simulink model "IntecoPhysicalOriginal"  (R2020b)
settings: Solver=ode5  StartTime=0.0  StopTime=9999  FixedStep=0.01  RelTol=1e-3  AbsTol=1e-6
libraries: simulink x2
settings Model: SimulationMode=external  ExtModeTrigDuration=12000  ExtModeTrigLevel=0.400000  Creator=jims  LastModifiedBy=Mark
settings SolverCC: AutoScaleAbsTol=off
settings DataIOCC: ExternalInput=[]  InitialState=[]  MaxDataPoints=5000  SaveFormat=Array  SignalLoggingSaveFormat=ModelDataLogs  SaveOutput=off  SaveTime=off  ReturnWorkspaceOutputs=off  SignalLoggingName=sigsOut
settings OptimizationCC: BooleanDataType=off  ExpressionDepthLimit=2147483647  InitFltsAndDblsToZero=on
settings DebuggingCC: SaveWithParameterizedLinksMsg=none  UnderspecifiedInitializationDetection=Classic  MergeDetectMultiDrivingBlocksExec=none  SignalResolutionControl=TryResolveAllWithWarning  MultiTaskDSMMsg=warning  MultiTaskCondExecSysMsg=none  IntegerOverflowMsg=none  FcnCallInpInsideContextMsg=warning  StateNameClashWarn=warning  SFUnexpectedBacktrackingDiag=warning  SFNoUnconditionalDefaultTransitionDiag=warning  SFExecutionAtInitializationDiag=none  IntegerSaturationMsg=none  ArithmeticOperatorsInVariantConditions=warning
settings ModelReferenceCC: PropagateSignalLabelsOutOfModel=off
settings SFSimCC: SimUseLocalCustomCode=off  CustomCodeUndefinedFunction=UseInterfaceOnly
settings RTWCC: Description=Simulink Desktop Real-Time  SystemTargetFile=sldrt.tlc  TemplateMakefile=sldrt.tmf  RTWUseLocalCustomCode=off  RTWCompilerOptimization=on
settings CodeAppCC: MaxIdLength=95  StateflowObjectComments=on
settings SimulinkDesktopRealTimeCC: TargetPreCompLibLocation=C:\Program Files\MATLAB\R2020b\toolbox\sldrt\lib\win64  TargetLangStandard=C89/C90 (ANSI)  SupportVariableSizeSignals=off
settings ConfigComp: CovMetricSettings=dw  CovSaveCumulativeToWorkspaceVar=on  CovSaveSingleToWorkspaceVar=on  CovExternalEMLEnable=off

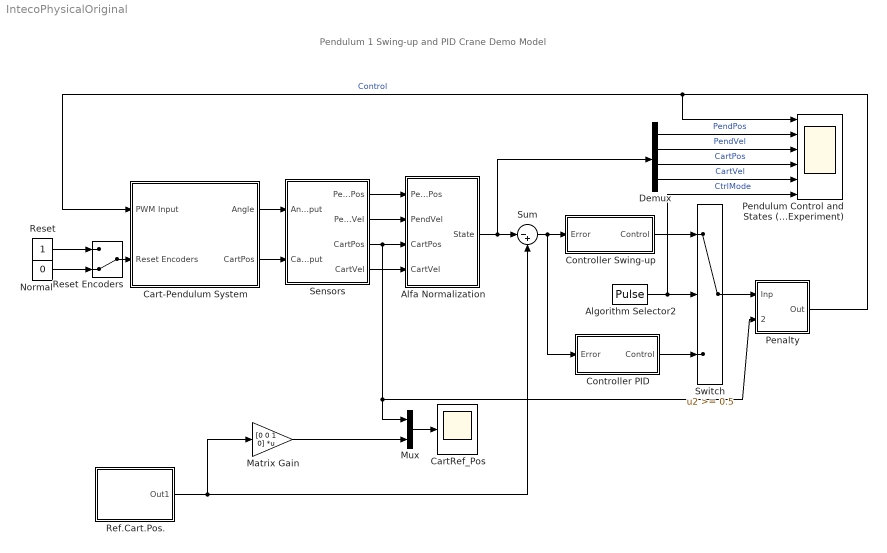
== system IntecoPhysicalOriginal ==
  note: Pendulum 1
      | Swing-up and PID Crane Demo Model
  Alfa Normalization : Subsystem  mask(Choose mode:){pos=Inverted Pendulum}
      mask prompts: pos "Choose mode:"
      mask TypeOptions pos: Inverted Pendulum | Crane Controller
  Algorithm Selector2 : DiscretePulseGenerator  PulseType=Time based  Period=60  PulseWidth=85  SampleTime=0.01
  Cart-Pendulum System : Subsystem  mask{BaseAddress=61184, T0=0.01}
      mask prompts: BaseAddress "Base Address:"; T0 "Sampling Period:"
      mask Display: plot( [0.725 0.725], [1.05 0.375], 0.725+0.05*sin([0:0.5:7]), 0.325+0.05*cos([0:0.5:7]), [-0.3 -0.3], [-0.3 -0.3], [1.8 1.8], [1.8 1.8], [0.1 1.4], [0.95 0.95], [0.1 1.4], [0.92 0.92], [0.65 0.8], [1 1], [0.65 0.8], [1.1 1.1], [0.65 0.65], [1.1 1], [0.8 0.8], [1 1.1] )
  CartRef_Pos : Scope
  Controller PID : Subsystem  mask{Cart_PID=[ -0.8 -0.0 -0.05], Pend_PID=[-1 0 -0.0 ], Umax=0.5, zone=1.3, Friction=0.05, T0=0.01}
      mask prompts: Cart_PID "Cart PID parameters [Kp, Ki, Kd]:"; Pend_PID "Pendulum PID parameters [Kp, Ki, Kd]:"; Umax "Maximum control value:"; zone "Stabilisation zone [rad]:"; Friction "Friction compensation:"; T0 "Sample time:"
  Controller Swing-up : Subsystem
  Demux : Demux
      settings: DisplayOption=none
  Matrix Gain : Gain  Gain=[0 0 1 0]  Multiplication=Matrix(K*u)  SaturateOnIntegerOverflow=on  OutDataTypeStr=Inherit: Same as input  ParamDataTypeStr=Inherit: Same as input
  Mux : Mux  Inputs=2
  Normal : Constant  Value=0
  Penalty : Subsystem
  Pendulum Control and States (Experiment) : Scope  NumInputPorts=6
  Ref.Cart.Pos. : Subsystem  mask{Sine=on, Square=off, Sawtooth=off, Amplitude=0., Frequency=0.05}
      mask Display: disp('Generator')
  Reset : Constant
  Reset Encoders : ManualSwitch  CurrentSetting=0
  Sensors : Subsystem  mask(PENDULUM Output){T0=0.01}
      mask prompts: T0 "Sample Time"
      mask help: PCL-812 PG Device Driver
  Sum : Sum  Inputs=|-+  InputSameDT=on  SaturateOnIntegerOverflow=on  OutDataTypeStr=Inherit: Same as first input
  Switch : Switch  Threshold=0.5  SaturateOnIntegerOverflow=on  InputSameDT=on
  wires:
  Reset Encoders/1 -> Cart-Pendulum System/2(Reset Encoders)
  Normal/1 -> Reset Encoders/2
  Reset/1 -> Reset Encoders/1
  Sensors/1(PendPos) -> Alfa Normalization/1(PendPos)
  Sensors/2(PendVel) -> Alfa Normalization/2(PendVel)
  Sensors/3(CartPos) -> Alfa Normalization/3(CartPos), Mux/1, Penalty/2(CartPos)
  Sensors/4(CartVel) -> Alfa Normalization/4(CartVel)
  Sum/1 -> Controller Swing-up/1(Error), Controller PID/1(Error)
  Ref.Cart.Pos./1(Out1) -> Sum/2, Matrix Gain/1
  Mux/1 -> CartRef_Pos/1
  Alfa Normalization/1(State) -> Sum/1, Demux/1
  Matrix Gain/1 -> Mux/2
  Penalty/1(Out) -> Pendulum Control and States (Experiment)/1, Cart-Pendulum System/1(PWM Input)  "Control"
  Algorithm Selector2/1 -> Switch/2, Pendulum Control and States (Experiment)/6  "CtrlMode"
  Controller Swing-up/1(Control) -> Switch/1
  Controller PID/1(Control) -> Switch/3
  Switch/1 -> Penalty/1(Inp)
  Demux/4 -> Pendulum Control and States (Experiment)/5  "CartVel"
  Demux/3 -> Pendulum Control and States (Experiment)/4  "CartPos"
  Demux/2 -> Pendulum Control and States (Experiment)/3  "PendVel"
  Demux/1 -> Pendulum Control and States (Experiment)/2  "PendPos"
  Cart-Pendulum System/1(Angle) -> Sensors/1(AngleInput)
  Cart-Pendulum System/2(CartPos) -> Sensors/2(CartPosInput)

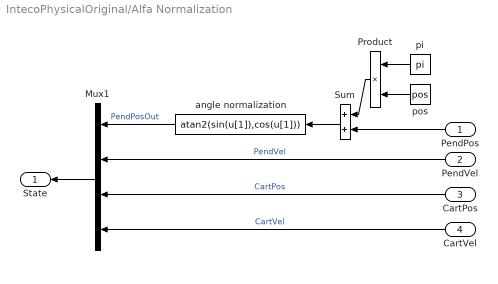
== system IntecoPhysicalOriginal/Alfa Normalization ==
  PendPos : Inport
  PendVel : Inport  Port=2
  CartPos : Inport  Port=3
  CartVel : Inport  Port=4
  Mux1 : Mux
  Product : Product  InputSameDT=on  SaturateOnIntegerOverflow=on  OutDataTypeStr=Inherit: Same as first input
  Sum : Sum  InputSameDT=on  SaturateOnIntegerOverflow=on  OutDataTypeStr=Inherit: Same as first input
  angle normalization : Fcn  Expr=atan2(sin(u[1]),cos(u[1]))
  pi : Constant  Value=pi
  pos : Constant  Value=pos
  State : Outport  InitialOutput=0
  wires:
  angle normalization/1 -> Mux1/1  "PendPosOut"
  PendVel/1 -> Mux1/2  "PendVel"
  CartVel/1 -> Mux1/4  "CartVel"
  CartPos/1 -> Mux1/3  "CartPos"
  Mux1/1 -> State/1
  Sum/1 -> angle normalization/1
  PendPos/1 -> Sum/2
  pi/1 -> Product/1
  pos/1 -> Product/2
  Product/1 -> Sum/1

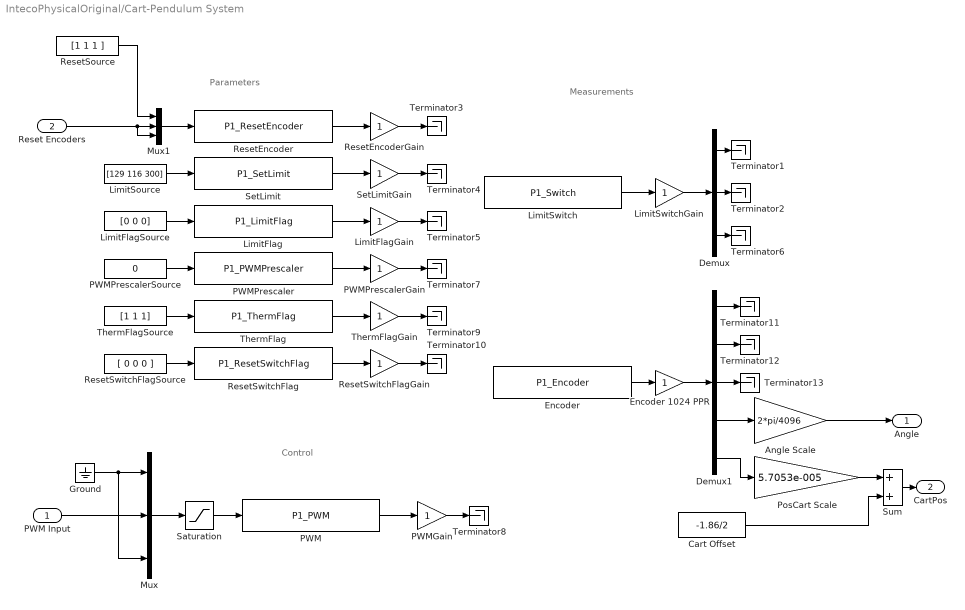
== system IntecoPhysicalOriginal/Cart-Pendulum System ==
  note: Measurements
  note: Control
  note: Parameters
  PWM Input : Inport
  Reset Encoders : Inport  Port=2
  Angle Scale : Gain  Gain=2*pi/4096  OutDataTypeStr=Inherit: Same as input  ParamDataTypeStr=Inherit: Same as input
  Cart Offset : Constant  Value=-1.86/2
  Demux : Demux  Outputs=3
      settings: DisplayOption=none
  Demux1 : Demux  Outputs=5
      settings: DisplayOption=none
  Encoder : S-Function  FunctionName=P1_Encoder  Parameters=BaseAddress, T0  SFunctionDeploymentMode=off  EnableBusSupport=off
  Encoder 1024 PPR : Gain  SaturateOnIntegerOverflow=on  OutDataTypeStr=Inherit: Same as input  ParamDataTypeStr=Inherit: Same as input
  Ground : Ground
  LimitFlag : S-Function  FunctionName=P1_LimitFlag  Parameters=BaseAddress, T0  SFunctionDeploymentMode=off  EnableBusSupport=off
  LimitFlagGain : Gain  SaturateOnIntegerOverflow=on  OutDataTypeStr=Inherit: Same as input  ParamDataTypeStr=Inherit: Same as input
  LimitFlagSource : Constant  Value=[0 0 0]
  LimitSource : Constant  Value=[129 116 300]
  LimitSwitch : S-Function  FunctionName=P1_Switch  Parameters=BaseAddress, T0  SFunctionDeploymentMode=off  EnableBusSupport=off
  LimitSwitchGain : Gain  SaturateOnIntegerOverflow=on  OutDataTypeStr=Inherit: Same as input  ParamDataTypeStr=Inherit: Same as input
  Mux : Mux  Inputs=3
  Mux1 : Mux  Inputs=[3 1 1]
  PWM : S-Function  FunctionName=P1_PWM  Parameters=BaseAddress, T0  SFunctionDeploymentMode=off  EnableBusSupport=off
  PWMGain : Gain  SaturateOnIntegerOverflow=on  OutDataTypeStr=Inherit: Same as input  ParamDataTypeStr=Inherit: Same as input
  PWMPrescaler : S-Function  FunctionName=P1_PWMPrescaler  Parameters=BaseAddress, T0  SFunctionDeploymentMode=off  EnableBusSupport=off
  PWMPrescalerGain : Gain  SaturateOnIntegerOverflow=on  OutDataTypeStr=Inherit: Same as input  ParamDataTypeStr=Inherit: Same as input
  PWMPrescalerSource : Constant  Value=0
  PosCart Scale : Gain  Gain=5.7053e-005  OutDataTypeStr=Inherit: Same as input  ParamDataTypeStr=Inherit: Same as input
  ResetEncoder : S-Function  FunctionName=P1_ResetEncoder  Parameters=BaseAddress, T0  SFunctionDeploymentMode=off  EnableBusSupport=off
  ResetEncoderGain : Gain  SaturateOnIntegerOverflow=on  OutDataTypeStr=Inherit: Same as input  ParamDataTypeStr=Inherit: Same as input
  ResetSource : Constant  Value=[1 1 1 ]
  "ResetSwitchFlag " : S-Function  FunctionName=P1_ResetSwitchFlag  Parameters=BaseAddress, T0  SFunctionDeploymentMode=off  EnableBusSupport=off
  ResetSwitchFlagGain : Gain  SaturateOnIntegerOverflow=on  OutDataTypeStr=Inherit: Same as input  ParamDataTypeStr=Inherit: Same as input
  ResetSwitchFlagSource : Constant  Value=[ 0 0 0 ]
  Saturation : Saturate
  SetLimit : S-Function  FunctionName=P1_SetLimit  Parameters=BaseAddress, T0  SFunctionDeploymentMode=off  EnableBusSupport=off
  SetLimitGain : Gain  SaturateOnIntegerOverflow=on  OutDataTypeStr=Inherit: Same as input  ParamDataTypeStr=Inherit: Same as input
  Sum : Sum  InputSameDT=on  SaturateOnIntegerOverflow=on  OutDataTypeStr=Inherit: Same as first input
  Terminator{1..13} (13 alike) : Terminator
  "ThermFlag " : S-Function  FunctionName=P1_ThermFlag  Parameters=BaseAddress, T0  SFunctionDeploymentMode=off  EnableBusSupport=off
  ThermFlagGain : Gain  SaturateOnIntegerOverflow=on  OutDataTypeStr=Inherit: Same as input  ParamDataTypeStr=Inherit: Same as input
  ThermFlagSource : Constant  Value=[1 1 1]
  Angle : Outport
  CartPos : Outport  Port=2
  wires:
  Demux1/1 -> Terminator11/1
  Demux1/2 -> Terminator12/1
  Demux1/3 -> Terminator13/1
  Demux1/4 -> Angle Scale/1
  Demux1/5 -> PosCart Scale/1
  Angle Scale/1 -> Angle/1
  Demux/3 -> Terminator6/1
  Demux/2 -> Terminator2/1
  Demux/1 -> Terminator1/1
  LimitSwitchGain/1 -> Demux/1
  LimitSwitch/1 -> LimitSwitchGain/1
  Ground/1 -> Mux/1, Mux/3
  PWM Input/1 -> Mux/2
  ResetSwitchFlagGain/1 -> Terminator10/1
  ThermFlagGain/1 -> Terminator9/1
  PWMPrescalerGain/1 -> Terminator7/1
  LimitFlagGain/1 -> Terminator5/1
  SetLimitGain/1 -> Terminator4/1
  ResetEncoderGain/1 -> Terminator3/1
  ResetSwitchFlagSource/1 -> "ResetSwitchFlag "/1
  ThermFlagSource/1 -> "ThermFlag "/1
  PWMPrescalerSource/1 -> PWMPrescaler/1
  LimitFlagSource/1 -> LimitFlag/1
  LimitSource/1 -> SetLimit/1
  "ResetSwitchFlag "/1 -> ResetSwitchFlagGain/1
  "ThermFlag "/1 -> ThermFlagGain/1
  PWMPrescaler/1 -> PWMPrescalerGain/1
  LimitFlag/1 -> LimitFlagGain/1
  SetLimit/1 -> SetLimitGain/1
  ResetEncoder/1 -> ResetEncoderGain/1
  PWMGain/1 -> Terminator8/1
  PWM/1 -> PWMGain/1
  Mux/1 -> Saturation/1
  Saturation/1 -> PWM/1
  Encoder/1 -> Encoder 1024 PPR/1
  Encoder 1024 PPR/1 -> Demux1/1
  Mux1/1 -> ResetEncoder/1
  ResetSource/1 -> Mux1/1
  Reset Encoders/1 -> Mux1/2, Mux1/3
  PosCart Scale/1 -> Sum/1
  Sum/1 -> CartPos/1
  Cart Offset/1 -> Sum/2

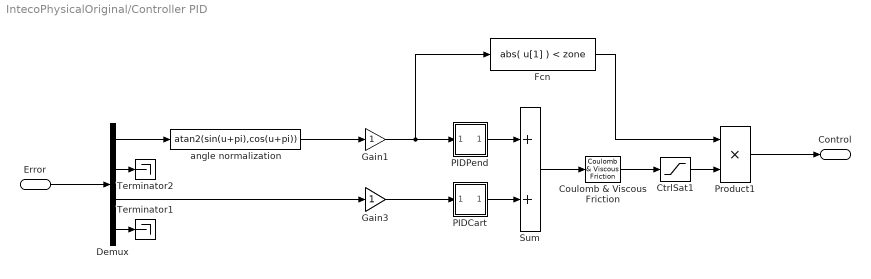
== system IntecoPhysicalOriginal/Controller PID ==
  Error : Inport
  Coulomb & Viscous Friction : simulink/Discontinuities/Coulomb & Viscous Friction  offset=Friction  gain=1
  CtrlSat1 : Saturate  UpperLimit=Umax  LowerLimit=-Umax
  Demux : Demux
      settings: DisplayOption=none
  Fcn : Fcn  Expr=abs( u[1] ) < zone
  Gain1 : Gain  SaturateOnIntegerOverflow=on  OutDataTypeStr=Inherit: Same as input  ParamDataTypeStr=Inherit: Same as input
  Gain3 : Gain  SaturateOnIntegerOverflow=on  OutDataTypeStr=Inherit: Same as input  ParamDataTypeStr=Inherit: Same as input
  PIDCart : Subsystem  mask(PID(2) Controller){P=Cart_PID(1), I=Cart_PID(2), D=Cart_PID(3), T0=T0}
      mask prompts: P "Proportional:"; I "Integral:"; D "Derivative:"; T0 "Sample Time:"
      mask help:
      | Enter Proportional(P), Integral(I), and Derivative(D) and divisor (N) terms.
      | P+I/s+Ds/(1/Ns+1)
      mask Help: This block implements a PID controller where parameters are entered for the Proportional, Integral and Derivative and divisor terms. Unmask this block to see how it works. The derivative term is implemented using an s/(s/N +1)  transfer function block. Making N large can create a "stiff" system.
      mask Display: disp('PID')
  PIDPend : Subsystem  mask(PID(2) Controller){P=Pend_PID(1), I=Pend_PID(2), D=Pend_PID(3), T0=T0}
      mask prompts: P "Proportional:"; I "Integral:"; D "Derivative:"; T0 "Sample Time:"
      mask help:
      | Enter Proportional(P), Integral(I), and Derivative(D) and divisor (N) terms.
      | P+I/s+Ds/(1/Ns+1)
      mask Help: This block implements a PID controller where parameters are entered for the Proportional, Integral and Derivative and divisor terms. Unmask this block to see how it works. The derivative term is implemented using an s/(s/N +1)  transfer function block. Making N large can create a "stiff" system.
      mask Display: disp('PID')
  Product1 : Product  InputSameDT=on  SaturateOnIntegerOverflow=on  OutDataTypeStr=Inherit: Same as first input
  Sum : Sum  InputSameDT=on  SaturateOnIntegerOverflow=on  OutDataTypeStr=Inherit: Same as first input
  Terminator1 : Terminator
  Terminator2 : Terminator
  angle normalization : Fcn  Expr=atan2(sin(u+pi),cos(u+pi))
  Control : Outport  InitialOutput=0
  wires:
  Demux/4 -> Terminator1/1
  Demux/3 -> Gain3/1
  Demux/2 -> Terminator2/1
  Error/1 -> Demux/1
  Demux/1 -> angle normalization/1
  Gain1/1 -> Fcn/1, PIDPend/1(In_1)
  PIDPend/1(Out_1) -> Sum/1
  Sum/1 -> Coulomb & Viscous Friction/1
  Coulomb & Viscous Friction/1 -> CtrlSat1/1
  CtrlSat1/1 -> Product1/2
  Fcn/1 -> Product1/1
  Product1/1 -> Control/1
  Gain3/1 -> PIDCart/1(In_1)
  PIDCart/1(Out_1) -> Sum/2
  angle normalization/1 -> Gain1/1

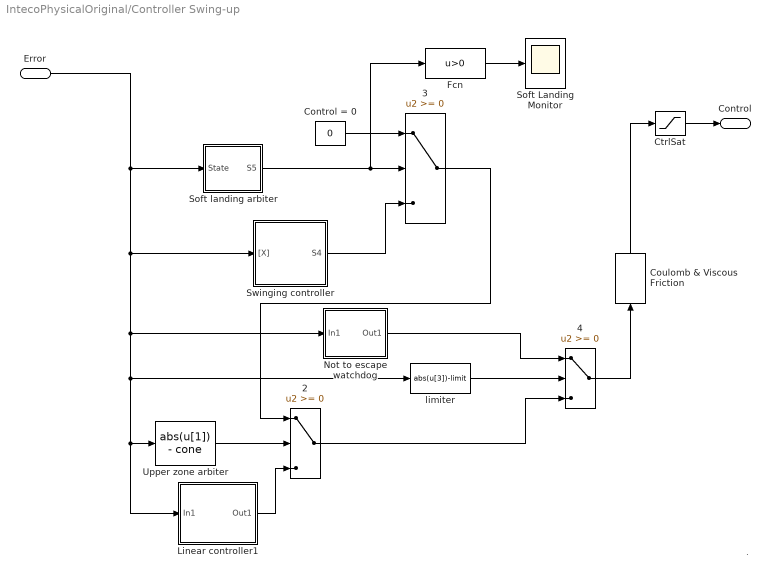
== system IntecoPhysicalOriginal/Controller Swing-up ==
  note: .
  Error : Inport
  2 : Switch  SaturateOnIntegerOverflow=on  InputSameDT=on
  3 : Switch  SaturateOnIntegerOverflow=on  InputSameDT=on
  4 : Switch  SaturateOnIntegerOverflow=on  InputSameDT=on
  Control = 0 : Constant  Value=0
  Coulomb & Viscous Friction : simulink/Discontinuities/Coulomb & Viscous Friction  offset=0.01  gain=1
  CtrlSat : Saturate  UpperLimit=1  LowerLimit=-1
  Fcn : Fcn  Expr=u>0
  Linear controller1 : Subsystem  mask(linear){umax1=0.2, K=[ 8 0.6 3.8 1.0 ]}
      mask prompts: umax1 "maximal control umax"; K "feedback K"
      mask Display: plot(0,0,100,100,[40,30,20],[87,85,80],[46,54,54,46,46],[90,90,80,80,90],[46,45,45,46,54,55,55,54,46],[78,80,90,91,91,90,80,78,78],[51,51,49,49],[78,10,10,78],[90,80,70,60],[70,80,85,88],[20,10],[80,70],[20,20,15],[73,80,80],[85,80,80],[80,80,74])
  Not to escape watchdog : Subsystem  mask{umax2=1}
      mask prompts: umax2 "maximal force"
      mask Display: plot(0,0,100,100,[20,40,40,20,20],[60,60,49,49,60],[56,59,40],[58,55,55],[56,59],[52,55],[38,13,13],[39,39,46],[46,13],[46,46],[23,23,24,22,24,24,22,23],[47,45,49,48,48,46,47,49],[36,35,34,34,37,34,36,35,36,37,35,34,35],[49,48,46,49,48,47,45,47,48,46,46,47,49],[22,22,24,24],[46,49,48,47])
  Soft Landing Monitor : Scope
  Soft landing arbiter : Subsystem  mask(Soft landing){k=8.5, R=0.3}
      mask prompts: k "k coefficient"; R "R value"
      mask help: Soft landing
      mask Display: plot(0,0,100,100,[14,20,20,14,14],[20,20,8,8,20],[40,35,35,40,40],[39,40,51,51,40],[60,55,55,56,60,60],[70,70,60,60,60,71],[74,74,80,80,74],[80,91,91,80,80])
  Swinging controller : Subsystem  mask(swing){umax=0.3}
      mask prompts: umax "maximal control umax"
      mask help: swing
      mask Display: plot(0,0,100,100,[20,20],[12,87],[93,90,90,93,7],[50,46,54,50,50],[20,22,18,20],[87,80,80,88],[80,80,75,75,71,71,65,65,60,60,49,49,40,40,20],[50,40,40,60,60,50,50,80,80,20,21,80,80,21,20])
  Upper zone arbiter : Fcn  Expr=abs(u[1]) - cone  mask(ZONE){cone=0.2}
      mask prompts: cone "width of stabilization zone [rad]"
      mask help: ZONE
      mask Display: plot(0,0,100,100,[40,60,80,83,80,60,40,20,17,20,40],[89,89,80,70,60,51,51,60,69,80,90],[83,50,17],[70,8,68])
  limiter : Fcn  Expr=abs(u[3])-limit  mask{limit=0.5}
      mask prompts: limit "rail limit"
      mask Display: plot(0,0,100,100,[10,90,90,10],[52,52,50,50],[30,30],[52,60],[70,68,68,70,70],[60,60,52,52,60],[30,32,32,30],[52,52,60,60])
  Control : Outport  InitialOutput=0
  wires:
  CtrlSat/1 -> Control/1
  Linear controller1/1(Out1) -> 2/3
  Upper zone arbiter/1 -> 2/2
  4/1 -> Coulomb & Viscous Friction/1
  Not to escape watchdog/1(Out1) -> 4/1
  limiter/1 -> 4/2
  Error/1 -> Not to escape watchdog/1(In1), Upper zone arbiter/1, Linear controller1/1(In1), limiter/1, Swinging controller/1("[X]"), Soft landing arbiter/1(State)
  Soft landing arbiter/1(S5) -> 3/2, Fcn/1
  Control = 0/1 -> 3/1
  Swinging controller/1(S4) -> 3/3
  3/1 -> 2/1
  2/1 -> 4/3
  Coulomb & Viscous Friction/1 -> CtrlSat/1
  Fcn/1 -> Soft Landing Monitor/1

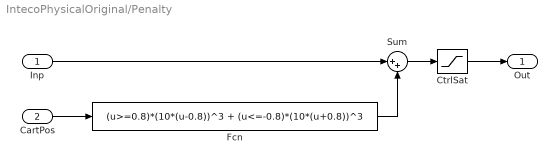
== system IntecoPhysicalOriginal/Penalty ==
  Inp : Inport
  CartPos : Inport  Port=2
  CtrlSat : Saturate  UpperLimit=0.4  LowerLimit=-0.4
  Fcn : Fcn  Expr=(u>=0.8)*(10*(u-0.8))^3 + (u<=-0.8)*(10*(u+0.8))^3
  Sum : Sum  Inputs=|++  InputSameDT=on  SaturateOnIntegerOverflow=on  OutDataTypeStr=Inherit: Same as first input
  Out : Outport
  wires:
  Inp/1 -> Sum/1
  Fcn/1 -> Sum/2
  CartPos/1 -> Fcn/1
  Sum/1 -> CtrlSat/1
  CtrlSat/1 -> Out/1

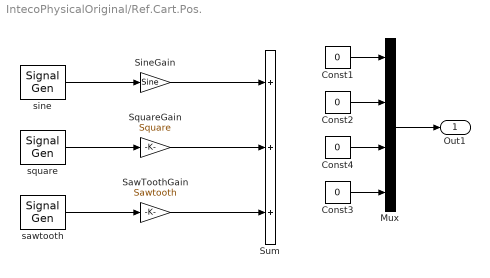
== system IntecoPhysicalOriginal/Ref.Cart.Pos. ==
  Const{1..4} (4 alike) : Constant  Value=0
  Mux : Mux
  SawToothGain : Gain  Gain=Sawtooth  SaturateOnIntegerOverflow=on  OutDataTypeStr=Inherit: Same as input  ParamDataTypeStr=Inherit: Same as input
  SineGain : Gain  Gain=Sine  SaturateOnIntegerOverflow=on  OutDataTypeStr=Inherit: Same as input  ParamDataTypeStr=Inherit: Same as input
  SquareGain : Gain  Gain=Square  SaturateOnIntegerOverflow=on  OutDataTypeStr=Inherit: Same as input  ParamDataTypeStr=Inherit: Same as input
  Sum : Sum  Inputs=+++  InputSameDT=on  SaturateOnIntegerOverflow=on  OutDataTypeStr=Inherit: Same as first input
  sawtooth : SignalGenerator  WaveForm=sawtooth  Amplitude=Amplitude  Frequency=Frequency
  sine : SignalGenerator  Amplitude=Amplitude  Frequency=Frequency
  square : SignalGenerator  WaveForm=square  Amplitude=Amplitude  Frequency=Frequency
  Out1 : Outport  InitialOutput=0
  wires:
  SawToothGain/1 -> Sum/3
  SquareGain/1 -> Sum/2
  SineGain/1 -> Sum/1
  sawtooth/1 -> SawToothGain/1
  square/1 -> SquareGain/1
  sine/1 -> SineGain/1
  Const1/1 -> Mux/1
  Const2/1 -> Mux/2
  Const3/1 -> Mux/4
  Mux/1 -> Out1/1
  Const4/1 -> Mux/3

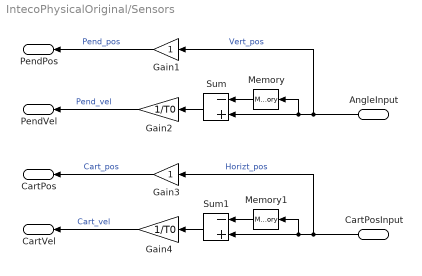
== system IntecoPhysicalOriginal/Sensors ==
  AngleInput : Inport
  CartPosInput : Inport  Port=2
  Gain1 : Gain  SaturateOnIntegerOverflow=on  OutDataTypeStr=Inherit: Same as input  ParamDataTypeStr=Inherit: Same as input
  Gain2 : Gain  Gain=1/T0  SaturateOnIntegerOverflow=on  OutDataTypeStr=Inherit: Same as input  ParamDataTypeStr=Inherit: Same as input
  Gain3 : Gain  SaturateOnIntegerOverflow=on  OutDataTypeStr=Inherit: Same as input  ParamDataTypeStr=Inherit: Same as input
  Gain4 : Gain  Gain=1/T0  SaturateOnIntegerOverflow=on  OutDataTypeStr=Inherit: Same as input  ParamDataTypeStr=Inherit: Same as input
  Memory : Memory
  Memory1 : Memory
  Sum : Sum  Inputs=-+  InputSameDT=on  SaturateOnIntegerOverflow=on  OutDataTypeStr=Inherit: Same as first input
  Sum1 : Sum  Inputs=-+  InputSameDT=on  SaturateOnIntegerOverflow=on  OutDataTypeStr=Inherit: Same as first input
  PendPos : Outport  InitialOutput=0
  PendVel : Outport  Port=2  InitialOutput=0
  CartPos : Outport  Port=3  InitialOutput=0
  CartVel : Outport  Port=4  InitialOutput=0
  wires:
  Gain4/1 -> CartVel/1  "Cart_vel"
  Sum1/1 -> Gain4/1
  Memory1/1 -> Sum1/1
  Sum/1 -> Gain2/1
  Memory/1 -> Sum/1
  CartPosInput/1 -> Memory1/1, Sum1/2, Gain3/1  "Horizt_pos"
  AngleInput/1 -> Memory/1, Sum/2, Gain1/1  "Vert_pos"
  Gain2/1 -> PendVel/1  "Pend_vel"
  Gain1/1 -> PendPos/1  "Pend_pos"
  Gain3/1 -> CartPos/1  "Cart_pos"

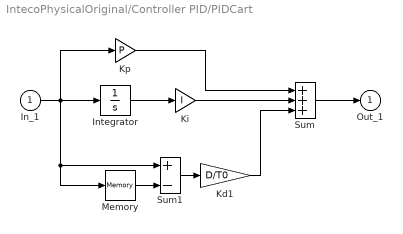
== system IntecoPhysicalOriginal/Controller PID/PIDCart ==
  In_1 : Inport
  Integrator : Integrator  LimitOutput=on  UpperSaturationLimit=1  LowerSaturationLimit=-1
  Kd1 : Gain  Gain=D/T0  SaturateOnIntegerOverflow=on  OutDataTypeStr=Inherit: Same as input  ParamDataTypeStr=Inherit: Same as input
  Ki : Gain  Gain=I  SaturateOnIntegerOverflow=on  OutDataTypeStr=Inherit: Same as input  ParamDataTypeStr=Inherit: Same as input
  Kp : Gain  Gain=P  SaturateOnIntegerOverflow=on  OutDataTypeStr=Inherit: Same as input  ParamDataTypeStr=Inherit: Same as input
  Memory : Memory
  Sum : Sum  Inputs=+++  InputSameDT=on  SaturateOnIntegerOverflow=on  OutDataTypeStr=Inherit: Same as first input
  Sum1 : Sum  Inputs=+-  InputSameDT=on  SaturateOnIntegerOverflow=on  OutDataTypeStr=Inherit: Same as first input
  Out_1 : Outport  InitialOutput=0
  wires:
  Ki/1 -> Sum/2
  Integrator/1 -> Ki/1
  In_1/1 -> Integrator/1, Kp/1, Memory/1, Sum1/1
  Sum/1 -> Out_1/1
  Kp/1 -> Sum/1
  Memory/1 -> Sum1/2
  Sum1/1 -> Kd1/1
  Kd1/1 -> Sum/3

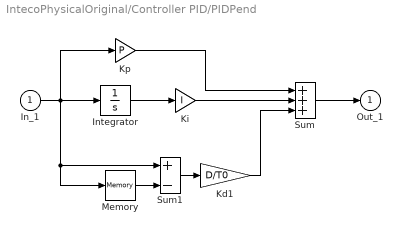
== system IntecoPhysicalOriginal/Controller PID/PIDPend ==
  In_1 : Inport
  Integrator : Integrator  LimitOutput=on  UpperSaturationLimit=1  LowerSaturationLimit=-1
  Kd1 : Gain  Gain=D/T0  SaturateOnIntegerOverflow=on  OutDataTypeStr=Inherit: Same as input  ParamDataTypeStr=Inherit: Same as input
  Ki : Gain  Gain=I  SaturateOnIntegerOverflow=on  OutDataTypeStr=Inherit: Same as input  ParamDataTypeStr=Inherit: Same as input
  Kp : Gain  Gain=P  SaturateOnIntegerOverflow=on  OutDataTypeStr=Inherit: Same as input  ParamDataTypeStr=Inherit: Same as input
  Memory : Memory
  Sum : Sum  Inputs=+++  InputSameDT=on  SaturateOnIntegerOverflow=on  OutDataTypeStr=Inherit: Same as first input
  Sum1 : Sum  Inputs=+-  InputSameDT=on  SaturateOnIntegerOverflow=on  OutDataTypeStr=Inherit: Same as first input
  Out_1 : Outport  InitialOutput=0
  wires:
  Kd1/1 -> Sum/3
  Sum1/1 -> Kd1/1
  Memory/1 -> Sum1/2
  Kp/1 -> Sum/1
  Sum/1 -> Out_1/1
  In_1/1 -> Sum1/1, Memory/1, Kp/1, Integrator/1
  Integrator/1 -> Ki/1
  Ki/1 -> Sum/2

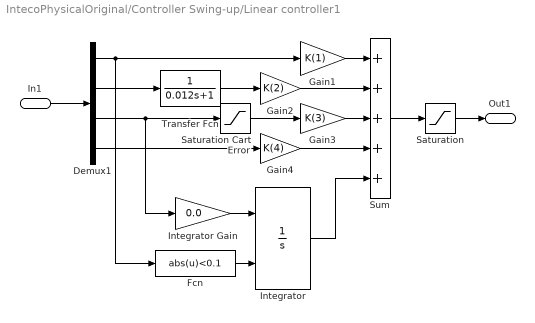
== system IntecoPhysicalOriginal/Controller Swing-up/Linear controller1 ==
  In1 : Inport
  Demux1 : Demux
      settings: DisplayOption=none
  Fcn : Fcn  Expr=abs(u)<0.1
  Gain1 : Gain  Gain=K(1)  SaturateOnIntegerOverflow=on  OutDataTypeStr=Inherit: Same as input  ParamDataTypeStr=Inherit: Same as input
  Gain2 : Gain  Gain=K(2)  SaturateOnIntegerOverflow=on  OutDataTypeStr=Inherit: Same as input  ParamDataTypeStr=Inherit: Same as input
  Gain3 : Gain  Gain=K(3)  SaturateOnIntegerOverflow=on  OutDataTypeStr=Inherit: Same as input  ParamDataTypeStr=Inherit: Same as input
  Gain4 : Gain  Gain=K(4)  SaturateOnIntegerOverflow=on  OutDataTypeStr=Inherit: Same as input  ParamDataTypeStr=Inherit: Same as input
  Integrator : Integrator  ExternalReset=rising  LimitOutput=on  UpperSaturationLimit=0.2  LowerSaturationLimit=-0.2
  Integrator Gain : Gain  Gain=0.0  SaturateOnIntegerOverflow=on  OutDataTypeStr=Inherit: Same as input  ParamDataTypeStr=Inherit: Same as input
  Saturation : Saturate  UpperLimit=umax1  LowerLimit=-umax1
  Saturation Cart Error : Saturate  UpperLimit=0.1  LowerLimit=-0.1
  Sum : Sum  Inputs=+++++  InputSameDT=on  SaturateOnIntegerOverflow=on  OutDataTypeStr=Inherit: Same as first input
  Transfer Fcn : TransferFcn  Denominator=[0.012 1]
  Out1 : Outport  InitialOutput=0
  wires:
  Saturation Cart Error/1 -> Gain3/1
  Integrator Gain/1 -> Integrator/1
  Fcn/1 -> Integrator/2
  Integrator/1 -> Sum/5
  Transfer Fcn/1 -> Gain2/1
  Demux1/1 -> Fcn/1, Gain1/1
  Saturation/1 -> Out1/1
  Gain1/1 -> Sum/1
  Gain2/1 -> Sum/2
  Demux1/2 -> Transfer Fcn/1
  Gain3/1 -> Sum/3
  Demux1/3 -> Saturation Cart Error/1, Integrator Gain/1
  Gain4/1 -> Sum/4
  Demux1/4 -> Gain4/1
  Sum/1 -> Saturation/1
  In1/1 -> Demux1/1

== system IntecoPhysicalOriginal/Controller Swing-up/Not to escape watchdog ==
  In1 : Inport
  Fcn : Fcn  Expr=-u[3]
  Gain : Gain  Gain=umax2  SaturateOnIntegerOverflow=on  OutDataTypeStr=Inherit: Same as input  ParamDataTypeStr=Inherit: Same as input
  Sign : Signum
  Out1 : Outport  InitialOutput=0
  wires:
  In1/1 -> Fcn/1
  Fcn/1 -> Sign/1
  Gain/1 -> Out1/1
  Sign/1 -> Gain/1

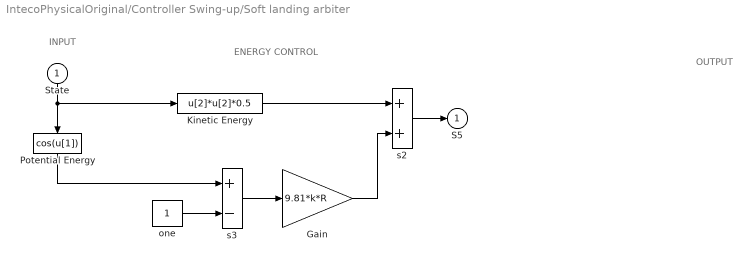
== system IntecoPhysicalOriginal/Controller Swing-up/Soft landing arbiter ==
  note: INPUT
  note: OUTPUT
  note: ENERGY CONTROL
  State : Inport
  Gain : Gain  Gain=9.81*k*R  SaturateOnIntegerOverflow=on  OutDataTypeStr=Inherit: Same as input  ParamDataTypeStr=Inherit: Same as input
  Kinetic Energy : Fcn  Expr=u[2]*u[2]*0.5
  Potential Energy : Fcn  Expr=cos(u[1])
  "one " : Constant
  s2 : Sum  InputSameDT=on  SaturateOnIntegerOverflow=on  OutDataTypeStr=Inherit: Same as first input
  s3 : Sum  Inputs=+-  InputSameDT=on  SaturateOnIntegerOverflow=on  OutDataTypeStr=Inherit: Same as first input
  S5 : Outport  InitialOutput=0
  wires:
  s2/1 -> S5/1
  State/1 -> Kinetic Energy/1, Potential Energy/1
  Gain/1 -> s2/2
  s3/1 -> Gain/1
  Kinetic Energy/1 -> s2/1
  "one "/1 -> s3/2
  Potential Energy/1 -> s3/1

== system IntecoPhysicalOriginal/Controller Swing-up/Swinging controller ==
  "[X]" : Inport
  abs(x1) : Fcn  Expr=u[2]*(abs(u[1])-pi/2)
  swing : Relay  OffOutputValue=-1
  umax : Gain  Gain=umax  SaturateOnIntegerOverflow=on  OutDataTypeStr=Inherit: Same as input  ParamDataTypeStr=Inherit: Same as input
  S4 : Outport  InitialOutput=0
  wires:
  abs(x1)/1 -> swing/1
  swing/1 -> umax/1
  "[X]"/1 -> abs(x1)/1
  umax/1 -> S4/1
